simulink model "eha_model_w_smc"  (R2015b)
settings: Solver=VariableStepAuto  StartTime=0.0  StopTime=10.0  RelTol=1e-3
values from neighbouring files (symbols this model uses):
  A = a    [rscale.m]
  B = b    [rscale.m]
  C = c    [rscale.m]
  K = k    [rscale.m]
  Nbar = Nu + K*Nx    [rscale.m]
undefined symbols (not defined in the file or in its folder): gaussian, L
libraries: simulink x1
settings Model: Creator=mathi  LastModifiedBy=Nicholas

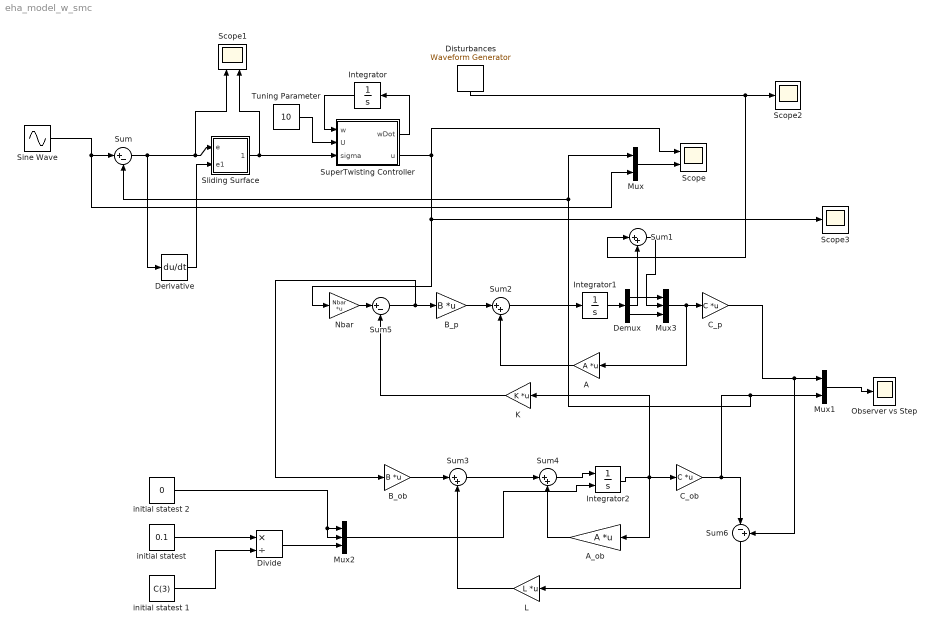
== system eha_model_w_smc ==
  A : Gain  Gain=A  Multiplication=Matrix(K*u)
  A_ob : Gain  Gain=A  Multiplication=Matrix(K*u)
  B_ob : Gain  Gain=B  Multiplication=Matrix(K*u)
  B_p : Gain  Gain=B  Multiplication=Matrix(K*u)
  C_ob : Gain  Gain=C  Multiplication=Matrix(K*u)
  C_p : Gain  Gain=C  Multiplication=Matrix(K*u)
  Demux : Demux  Outputs=3
  Derivative : Derivative
  Disturbances : simulink/Sources/Waveform Generator  OutMin=[]  OutMax=[]  OutDataTypeStr=double  SelectedSignal=1  Signals=gaussian(0,0,121313)  BlockNames=MultiportSwitch_d64598e6258c4fb  SampleTime=0.001
  Divide : Product  Inputs=*/
  Integrator : Integrator
  Integrator1 : Integrator
  Integrator2 : Integrator  InitialConditionSource=external  InitialCondition=[0 0 1/C(0)]
  K : Gain  Gain=K  Multiplication=Matrix(K*u)
  L : Gain  Gain=L  Multiplication=Matrix(K*u)
  Mux : Mux  Inputs=2
  Mux1 : Mux  Inputs=2
  Mux2 : Mux  Inputs=3
  Mux3 : Mux  Inputs=3
  Nbar : Gain  Gain=Nbar  Multiplication=Matrix(K*u)
  Observer vs Step : Scope
  Scope : Scope  NumInputPorts=2
  Scope1 : Scope  NumInputPorts=2
  Scope2 : Scope
  Scope3 : Scope
  Sine Wave : Sin  Frequency=2  SampleTime=0
  "Sliding Surface " : Subsystem
  Sum : Sum  Inputs=|+-
  Sum{1..4} (4 alike) : Sum  Inputs=|++
  Sum5 : Sum  Inputs=|+-
  Sum6 : Sum  Inputs=|-+
  SuperTwisting Controller : MATLAB Function  TreatAsAtomicUnit=on
  Tuning Parameter : Constant  Value=10
  "initial statest " : Constant  Value=0.1
  initial statest 1 : Constant  Value=C(3)
  initial statest 2 : Constant  Value=0
  wires:
  C_ob/1 -> Sum6/1, Mux/1, Sum/2, Mux1/2
  Mux/1 -> Scope/2
  "Sliding Surface "/1(Sigma) -> SuperTwisting Controller/3(sigma), Scope1/2
  SuperTwisting Controller/1(wDot) -> Integrator/1
  Integrator/1 -> SuperTwisting Controller/1(w)
  Tuning Parameter/1 -> SuperTwisting Controller/2(U)
  Disturbances/1 -> Sum1/1, Scope2/1
  Sum/1 -> "Sliding Surface "/1(e), Scope1/1, Derivative/1
  SuperTwisting Controller/2(u) -> Nbar/1, Scope3/1, Scope/1
  A/1 -> Sum2/2
  L/1 -> Sum3/2
  Sum3/1 -> Sum4/1
  A_ob/1 -> Sum4/2
  Sum4/1 -> Integrator2/1
  Integrator2/1 -> K/1, C_ob/1, A_ob/1
  B_ob/1 -> Sum3/1
  Mux1/1 -> Observer vs Step/1
  K/1 -> Sum5/2
  Sum5/1 -> B_ob/1, B_p/1
  Sum6/1 -> L/1
  Sine Wave/1 -> Sum/1, Mux/2
  Nbar/1 -> Sum5/1
  C_p/1 -> Sum6/2, Mux1/1
  Derivative/1 -> "Sliding Surface "/2(e1)
  "initial statest "/1 -> Divide/1
  initial statest 1/1 -> Divide/2
  Divide/1 -> Mux2/3
  initial statest 2/1 -> Mux2/2, Mux2/1
  Mux2/1 -> Integrator2/2
  Sum1/1 -> Mux3/2
  B_p/1 -> Sum2/1
  Demux/1 -> Mux3/1
  Demux/3 -> Mux3/3
  Demux/2 -> Sum1/2
  Integrator1/1 -> Demux/1
  Mux3/1 -> A/1, C_p/1
  Sum2/1 -> Integrator1/1

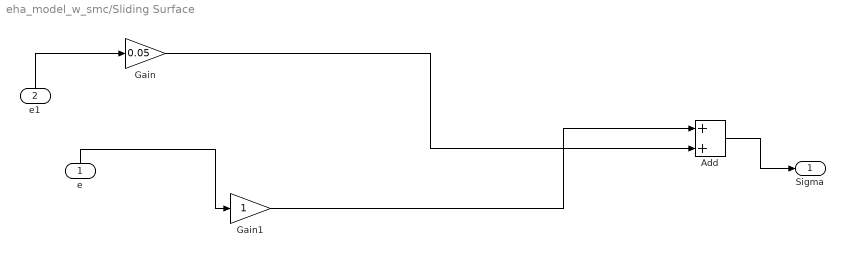
== system eha_model_w_smc/Sliding Surface  ==
  e : Inport
  e1 : Inport  Port=2
  Add : Sum
  Gain : Gain  Gain=0.05
  Gain1 : Gain
  Sigma : Outport
  wires:
  Add/1 -> Sigma/1
  e1/1 -> Gain/1
  Gain/1 -> Add/2
  e/1 -> Gain1/1
  Gain1/1 -> Add/1

== matlab function eha_model_w_smc/SuperTwisting Controller ==
  data: w input; U input; wDot output; u output; sigma input
function [wDot,u] = fcn(w,U,sigma)

lambda = sqrt(U);
W = 1.1*U;

u = lambda*sqrt(abs(sigma))*sign(sigma) + w;
 wDot = W*sign(sigma);
